simulink model "untitled"  (R2021a)
settings: Solver=VariableStepAuto  StartTime=0.0  StopTime=10.0  RelTol=1e-3
settings Model: Creator=VTX  LastModifiedBy=VTX

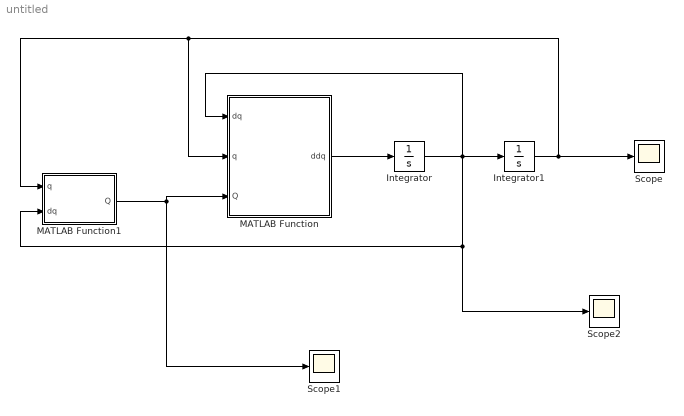
== system untitled ==
  Integrator : Integrator  InitialCondition=[0;0;pi/18]
  Integrator1 : Integrator  InitialCondition=[-pi/2;pi/6;0]
  MATLAB Function : MATLAB Function  TreatAsAtomicUnit=on
  MATLAB Function1 : MATLAB Function  TreatAsAtomicUnit=on
  Scope : Scope
  Scope1 : Scope
  Scope2 : Scope
  wires:
  MATLAB Function/1(ddq) -> Integrator/1
  Integrator/1 -> Scope2/1, MATLAB Function1/2(dq), MATLAB Function/1(dq), Integrator1/1
  Integrator1/1 -> Scope/1, MATLAB Function1/1(q), MATLAB Function/2(q)
  MATLAB Function1/1(Q) -> MATLAB Function/3(Q), Scope1/1

== matlab function untitled/MATLAB Function ==
  data: ddq output size=3; dq input size=3; q input size=3; Q input size=3
function ddq = fcn(dq,q,Q)
    q1 = q(1);
    q2 = q(2);
    q3 = q(3);
    
    l1 = 1;
    l2 = 1;
    l3 = 1;
    m1 = 1;
    m2 = 1;
    m3 = 1;
    P1 = 1;
    P2 = -0.72;

    %% Mass matrix
    M = [(m1 + m2 + m3)*l1^2 (m2 + m3)*l1*l2*cos(q2 - q1) m3*l1*l3*cos(q3 - q1); ...
    (m2 + m3)*l1*l2*cos(q2 - q1) (m2 + m3)*l2^2 m3*l1*l3*cos(q3 - q2); ...
    m3*l1*l3*cos(q3 - q1) m3*l1*l3*cos(q3 - q2) m3*l3^2];

    %% dq'*M_q(q)*dq
    dM_q1 = [0 (m2 + m3)*l1*l2*sin(q2 - q1) m3*l1*l3*sin(q3 - q1); ...
    (m2 + m3)*l1*l2*sin(q2 - q1) 0 0; ...
    m3*l1*l3*sin(q3 - q1) 0 0];

    dM_q2 = [0 -(m2 + m3)*l1*l2*sin(q2 - q1) 0; ...
    -(m2 + m3)*l1*l2*sin(q2 - q1) 0 m3*l1*l3*sin(q3 - q2); ...
    0 m3*l1*l3*sin(q3 - q2) 0];

    dM_q3 = [0 0 -m3*l1*l3*sin(q3 - q1); ...
    0 0 -m3*l1*l3*sin(q3 - q2); ...
    -m3*l1*l3*sin(q3 - q1) -m3*l1*l3*sin(q3 - q2) 0];

    Matrix = [dq'*dM_q1*dq;dq'*dM_q2*dq;dq'*dM_q3*dq];

    %% dM
    dM11 = 0;
    dM12 = [(m2 + m3)*l1*l2*sin(q2 - q1) -(m2 + m3)*l1*l2*sin(q2 - q1) 0]*dq;
    dM13 = [m3*l1*l3*sin(q3 - q1) 0 -m3*l1*l3*sin(q3 - q1)]*dq;

    dM21 = [(m2 + m3)*l1*l2*sin(q2 - q1) -(m2 + m3)*l1*l2*sin(q2 - q1) 0]*dq;
    dM22 = 0;
    dM23 = [0 m3*l1*l3*sin(q3 - q2) -m3*l1*l3*sin(q3 - q2)]*dq;

    dM31 = [m3*l1*l3*sin(q3 - q1) 0 -m3*l1*l3*sin(q3 - q1)]*dq;
    dM32 = [0 m3*l1*l3*sin(q3 - q2) -m3*l1*l3*sin(q3 - q2)]*dq;
    dM33 = 0;

    dM = [dM11 dM12 dM13;dM21 dM22 dM23;dM31 dM32 dM33];


    ddq = inv(M)*(-dM*dq + 1/2*Matrix + Q);
end

== matlab function untitled/MATLAB Function1 ==
  data: q input; dq input; Q output
function Q = fcn(q,dq)
    q1 = q(1);
    q2 = q(2);
    q3 = q(3);
    
    l1 = 1;
    l2 = 1;
    l3 = 1;
    m1 = 1;
    m2 = 1;
    m3 = 1;
    P1 = 1;
    P2 = -0.72;

    %% Mass matrix
    M = [(m1 + m2 + m3)*l1^2 (m2 + m3)*l1*l2*cos(q2 - q1) m3*l1*l3*cos(q3 - q1); ...
    (m2 + m3)*l1*l2*cos(q2 - q1) (m2 + m3)*l2^2 m3*l1*l3*cos(q3 - q2); ...
    m3*l1*l3*cos(q3 - q1) m3*l1*l3*cos(q3 - q2) m3*l3^2];

    Q = -P1*dq
    %Q = -P2*M*dq;
end
